simulink model "wireless_dynamic21aMATLAB"  (R2021a)
settings: Solver=FixedStepDiscrete  StartTime=0.0  StopTime=0.1  MaxStep=1e-6  RelTol=1e-3
undefined symbols (not defined in the file): DiscIntNeverNeededParam, Ion, Lithium
libraries: spsSeriesRLCBranchLib x4, spsDiodeLib x4, spsIGBTDiodeLib x4, spsCurrentMeasurementLib x2, spsBatteryLib x1, spsGroundLib x1, spsThreePhaseProgrammableVoltageSourceLib x1, spsUniversalBridgeLib x1, spsVoltageMeasurementLib x1, spspowerguiLib x1, spsMultiWindingTransformerLib x1, spsTriangleGeneratorLib x1
settings Model: Creator=Lenovo  LastModifiedBy=SHREYAS.D
settings SolverCC: AlgebraicLoopSolver=LineSearch
settings DataIOCC: ReturnWorkspaceOutputs=off
settings DebuggingCC: AlgebraicLoopMsg=none  ArithmeticOperatorsInVariantConditions=warning
settings SFSimCC: SimUseLocalCustomCode=off  CustomCodeUndefinedFunction=UseInterfaceOnly
settings RTWCC: RTWUseLocalCustomCode=off  DLArmComputeVersion=20.02.1
settings CodeAppCC: StateflowObjectComments=on
settings SimscapeCC: SimscapeNormalizeSystem=off

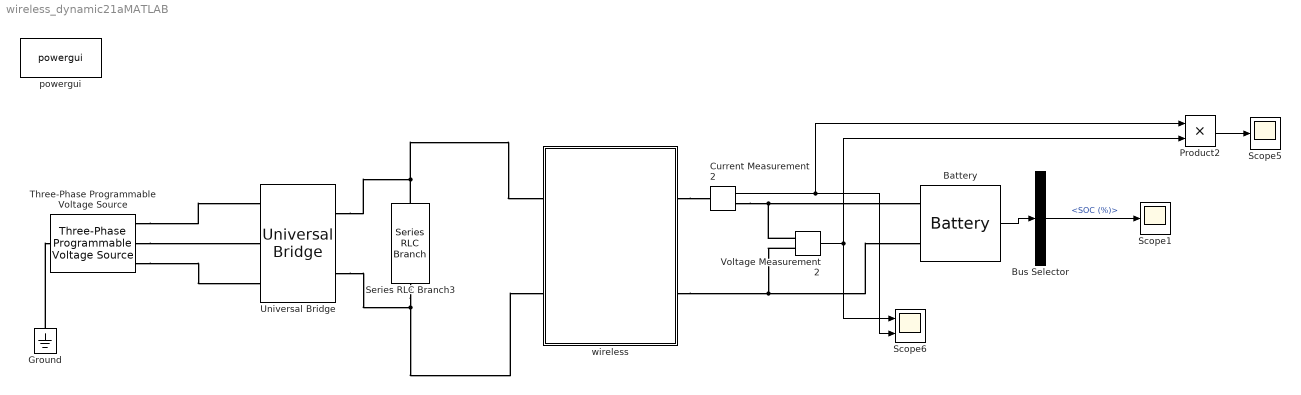
== system wireless_dynamic21aMATLAB ==
  Battery : spsBatteryLib/Battery  BatType=Lithium-Ion  ShowTempParam=off  ThermalPreset=no  ShowAgeParam=off  NomV=60  NomQ=300  SOC=80  Batt_Tr=30  PresetModel=on  MaxQ=300  MinV=45  FullV=69.8392  Dis_rate=130.4348  R=0.002  Normal_OP=271.3043  expZone="[64.8232      14.7391]"  current=[6.5 13 32.5]  Units=Time  Tci=20  NomT=20  T2=-30  MaxQ2=4.8  FullV2=7.1  Normal_OP2=5.655  expZone2="[6.58           1]"  Rca=0.6  ti=2000  Dp=0  Neq0=0  Tsim=1e6  Ta1=25  Qeol=5.4*0.9  Reol=0.013333*1.2  Char_age=[2.3478, 3]  Dis_age=[2.3478, 10]  N1=1500  N2=10500  N3=1000  N4=1400  Ta2=45  N5=950
  Bus Selector : BusSelector  OutputSignals=SOC (%)
  Current Measurement2 : spsCurrentMeasurementLib/Current Measurement  PhasorSimulation=off  OutputType=Complex  PSBequivalent=0
  Ground : spsGroundLib/Ground  LConnTagsString=a
  Product2 : Product
  Scope1 : Scope
  Scope5 : Scope
  Scope6 : Scope  NumInputPorts=2
  Series RLC Branch3 : spsSeriesRLCBranchLib/Series RLC Branch  LConnTagsString=__new0  RConnTagsString=__new0  BranchType=C  Resistance=0.001  Inductance=1e-3  SetiL0=off  InitialCurrent=0  Capacitance=2000e-6  Setx0=off  InitialVoltage=90  Measurements=None
  Three-Phase Programmable Voltage Source : spsThreePhaseProgrammableVoltageSourceLib/Three-Phase Programmable Voltage Source  PositiveSequence="[440  0 50]"  VariationEntity=None  VariationType=Table of time-amplitude pairs  VariationTypeAlt=Step  VariationStep=0.5  VariationRate=10  VariationMagnitude=0.3  VariationFrequency=2  VariationTiming=[1 2]  VariationPhaseA=off  Amplitudes=[1 0.8 1.2 1.0]  TimeValues=[0 0.1 0.15 0.2]  HarmonicGeneration=off  HarmonicA=[3 0.2 -25 0]  HarmonicB=[2 0.15 35 2]  Timing="[0.05  3]"  BusType=swing  Pref=0  Qref=0  Qmin=-inf  Qmax=inf
  Universal Bridge : spsUniversalBridgeLib/Universal Bridge  Arms=3  SnubberResistance=1e5  SnubberCapacitance=inf  Device=Diodes  Ron=1e-3  Lon=0  ForwardVoltages="[  0  0  ]"  ForwardVoltage=0  GTOparameters=[ 10e-6 , 20e-6 ]  IGBTparameters=[ 1e-6 , 2e-6 ]  Measurements=None  Measurements_2=None  converterType=Rectifier
  Voltage Measurement2 : spsVoltageMeasurementLib/Voltage Measurement  PhasorSimulation=off  OutputType=Complex  PSBequivalent=0
  powergui : spspowerguiLib/powergui  Priority=1  SimulationMode=Discrete  SampleTime=1e-6  frequency=60  Iterations=50  frequencyindice=0  Pbase=100e6  ErrMax=1e-4  UnitsV=kV  UnitsW=MW  buscounter=0  FunctionMessages=off  echomessages=off  EnableUseOfTLC=off  CurrentSourceSwitches=off  DisableSnubberDevices=off  DisableRonSwitches=off  DisableVfSwitches=off  DisplayEquations=off  AutomaticDiscreteSolvers=off  SolverType=Tustin/Backward Euler (TBE)  Interpol=off  ExternalGateDelay=off  methode=off  Ts=100  x0status=blocks  SPID=on  SwTol=0  HookPort=off  NonlinearTolerance=1e-4  nMaxIteration=100  ContinueOnMaxIteration=off  RestoreLinks=warning  ResistiveCurrentMeasurement=off  Frange=[0:2:500]  Ylog=off  Xlog=on  ShowGrid=off  save=off  variable=ZData  structure=0  ZoomFFT=off  StartTime=0.0  cycles=1  DisplayStyle=1  fundamental=60  FreqAxis=off  MaxFrequency=1000  frequencyindicesteady=1  RmsSteady=1  display=off
  wireless : Subsystem
  wires:
  Battery/1 -> Bus Selector/1
  Bus Selector/1 -> Scope1/1  "<SOC (%)>"
  Product2/1 -> Scope5/1
  Current Measurement2/1 -> Scope6/2, Product2/1
  Voltage Measurement2/1 -> Scope6/1, Product2/2
  connections:
  wireless/RConn2 -- Voltage Measurement2/LConn2 -- Battery/LConn2
  wireless/RConn1 -- Current Measurement2/LConn1
  Current Measurement2/RConn1 -- Voltage Measurement2/LConn1 -- Battery/LConn1
  Universal Bridge/RConn1 -- wireless/LConn1 -- Series RLC Branch3/LConn1
  Universal Bridge/RConn2 -- wireless/LConn2 -- Series RLC Branch3/RConn1
  Three-Phase Programmable Voltage Source/RConn1 -- Universal Bridge/LConn1
  Three-Phase Programmable Voltage Source/RConn2 -- Universal Bridge/LConn2
  Three-Phase Programmable Voltage Source/RConn3 -- Universal Bridge/LConn3
  Ground/LConn1 -- Three-Phase Programmable Voltage Source/LConn1

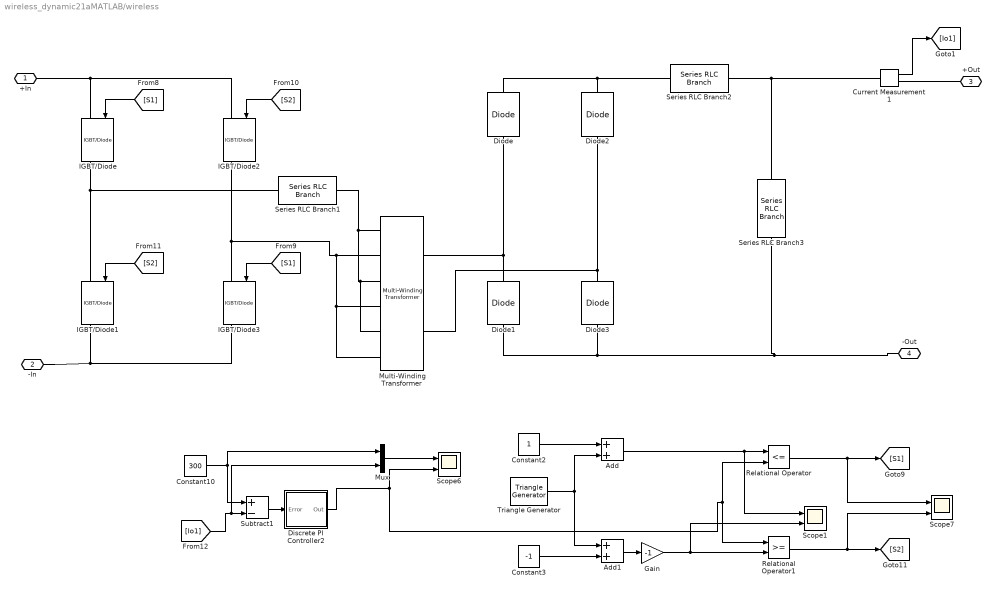
== system wireless_dynamic21aMATLAB/wireless ==
  Add : Sum
  Add1 : Sum
  Constant10 : Constant  Value=300
  Constant2 : Constant
  Constant3 : Constant  Value=-1
  Current Measurement1 : spsCurrentMeasurementLib/Current Measurement  PhasorSimulation=off  OutputType=Complex  PSBequivalent=0
  Diode{,1..3} (4 alike) : spsDiodeLib/Diode  Ron=0.001  Lon=0  Vf=0.8  IC=0  UseSnubber=0  Rs=500  Cs=250e-9  Measurements=off
  Discrete PI Controller2 : Subsystem  AncestorBlock=|  DialogController=POWERSYS.PowerSysDialog  mask(Discrete PI Controller){Kp=0.2, Ki=0.2, Par_Limits=[0.81 0], Init=0, Ts=1e-6}
      | powerlib_extras/Discrete 
      | Control Blocks/Discrete
      | PI Controller
      mask prompts: Kp "Proportional gain (Kp):"; Ki "Integral gain (Ki):"; Par_Limits "Output limits: [ Upper   Lower ]"; Init "Output initial value:"; Ts "Sample time:"
      mask help: This block implements a discrete PI controller.
      mask init:
      | UpperLimit=Par_Limits(1);
      | LowerLimit=Par_Limits(2);
      | power_initmask();
      mask Help: This block is part of a subset of blocks in the Extras library that does not have documentation associated with it, other than the block mask description.
      mask Display: disp('PI');
  Gain : Gain  Gain=-1
  IGBT/Diode{,1..3} (4 alike) : spsIGBTDiodeLib/IGBT//Diode  Ron=1e-3  Rs=1e5  Cs=inf  Measurements=on
  Multi-Winding Transformer : spsMultiWindingTransformerLib/Multi-Winding Transformer  LeftWindings=3  RightWindings=1  TappedWindings=no taps  NumberOfTaps=2  SetSaturation=off  Hysteresis=off  DataFile='hysteresis.mat'  Measurements=None  UNITS=SI  NominalPower=[20e3 20000]  NominalVoltages="[ 600  100  200 120 ]"  WindingResistances=[0.18 0.005 0.005 0.0072]  WindingInductances=[6.1879e-07 1.5915e-07 1.5915e-07 2.2918e-07]  Rm=1800  Lm=0.014324  Saturation=[0 0;0.056566 0.0081028;23.57 0.010264]  BreakLoop=off  DiscreteSolver=Trapezoidal iterative  DataType=on  InitialFlux=0  TransfoNumber=1
      settings: SourceProductBaseCode=PS
  Mux : Mux  Inputs=2
  Relational Operator : RelationalOperator  Operator=<=  OutDataTypeStr=boolean  RndMeth=Simplest
  Relational Operator1 : RelationalOperator  OutDataTypeStr=boolean  RndMeth=Simplest
  Scope1 : Scope  NumInputPorts=2
  Scope6 : Scope  NumInputPorts=2
  Scope7 : Scope  NumInputPorts=2
  Series RLC Branch1 : spsSeriesRLCBranchLib/Series RLC Branch  LConnTagsString=__new0  RConnTagsString=__new0  BranchType=L  Resistance=1  Inductance=0.31e-6  SetiL0=off  InitialCurrent=0  Capacitance=2000000e-6  Setx0=on  InitialVoltage=90  Measurements=None
  Series RLC Branch2 : spsSeriesRLCBranchLib/Series RLC Branch  LConnTagsString=__new0  RConnTagsString=__new0  BranchType=L  Resistance=1  Inductance=6.87e-6  SetiL0=off  InitialCurrent=0  Capacitance=2000000e-6  Setx0=on  InitialVoltage=90  Measurements=None
  Series RLC Branch3 : spsSeriesRLCBranchLib/Series RLC Branch  LConnTagsString=__new0  RConnTagsString=__new0  BranchType=C  Resistance=0.001  Inductance=1e-3  SetiL0=off  InitialCurrent=0  Capacitance=2000e-6  Setx0=off  InitialVoltage=90  Measurements=None
  Subtract1 : Sum  Inputs=+-
  Triangle Generator : spsTriangleGeneratorLib/Triangle Generator  Freq=20e3  Phase=0  Ts=0
  +In : PMIOPort  Side=Left
  -In : PMIOPort  Port=2  Side=Left
  +Out : PMIOPort  Port=3  Side=Right
  -Out : PMIOPort  Port=4  Side=Right
  wires:
  [S1] -> IGBT/Diode3/1
  [S1] -> IGBT/Diode/1
  [S2] -> IGBT/Diode2/1
  [S2] -> IGBT/Diode1/1
  Constant10/1 -> Mux/1, Subtract1/1
  [Io1] -> Subtract1/2, Mux/2
  Subtract1/1 -> Discrete PI Controller2/1(Error)
  Add1/1 -> Gain/1
  Mux/1 -> Scope6/1
  Relational Operator1/1 -> Scope7/2, [S2]
  Relational Operator/1 -> Scope7/1, [S1]
  Discrete PI Controller2/1(Out) -> Relational Operator1/1, Relational Operator/2, Scope6/2
  Add/1 -> Scope1/1, Relational Operator/1
  Triangle Generator/1 -> Add1/1, Add/2
  Constant2/1 -> Add/1
  Constant3/1 -> Add1/2
  Gain/1 -> Scope1/2, Relational Operator1/2
  Current Measurement1/1 -> [Io1]
  connections:
  IGBT/Diode/RConn1 -- IGBT/Diode1/LConn1 -- Series RLC Branch1/LConn1
  IGBT/Diode2/RConn1 -- Multi-Winding Transformer/LConn6 -- Multi-Winding Transformer/LConn4 -- Multi-Winding Transformer/LConn2 -- IGBT/Diode3/LConn1
  IGBT/Diode3/RConn1 -- IGBT/Diode1/RConn1 -- -In/RConn1
  IGBT/Diode2/LConn1 -- +In/RConn1 -- IGBT/Diode/LConn1
  Series RLC Branch1/RConn1 -- Multi-Winding Transformer/LConn5 -- Multi-Winding Transformer/LConn3 -- Multi-Winding Transformer/LConn1
  -Out/RConn1 -- Series RLC Branch3/RConn1 -- Diode3/LConn1 -- Diode1/LConn1
  Diode1/RConn1 -- Diode/LConn1 -- Multi-Winding Transformer/RConn1
  Diode3/RConn1 -- Diode2/LConn1 -- Multi-Winding Transformer/RConn2
  Diode2/RConn1 -- Diode/RConn1 -- Series RLC Branch2/LConn1
  Series RLC Branch2/RConn1 -- Current Measurement1/LConn1 -- Series RLC Branch3/LConn1
  Current Measurement1/RConn1 -- +Out/RConn1

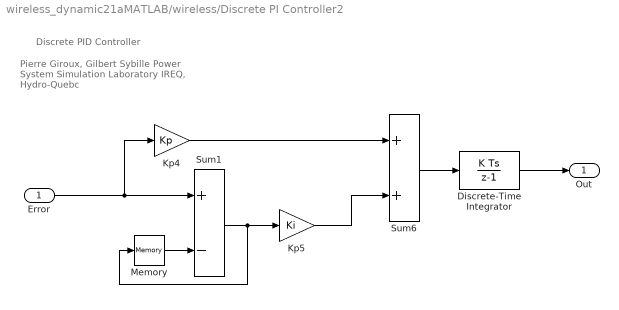
== system wireless_dynamic21aMATLAB/wireless/Discrete PI Controller2 ==
  note: Discrete PID Controller
  note: Pierre Giroux, Gilbert Sybille
      | Power System Simulation Laboratory
      | IREQ, Hydro-Quebc
  Error : Inport  SampleTime=Ts
  Discrete-Time Integrator : DiscreteIntegrator  InitialCondition=Init  SampleTime=Ts  LimitOutput=on  UpperSaturationLimit=UpperLimit  LowerSaturationLimit=LowerLimit  ICPrevOutput=DiscIntNeverNeededParam  ICPrevScaledInput=DiscIntNeverNeededParam
  Kp4 : Gain  Gain=Kp  SaturateOnIntegerOverflow=on  SampleTime=Ts  OutDataTypeStr=Inherit: Same as input  ParamDataTypeStr=Inherit: Same as input
  Kp5 : Gain  Gain=Ki  SaturateOnIntegerOverflow=on  SampleTime=Ts  OutDataTypeStr=Inherit: Same as input  ParamDataTypeStr=Inherit: Same as input
  Memory : Memory
  Sum1 : Sum  Inputs=+-  InputSameDT=on  SaturateOnIntegerOverflow=on  SampleTime=Ts  OutDataTypeStr=Inherit: Same as first input
  Sum6 : Sum  InputSameDT=on  SaturateOnIntegerOverflow=on  SampleTime=Ts  OutDataTypeStr=Inherit: Same as first input
  Out : Outport  SampleTime=Ts  InitialOutput=0
  wires:
  Sum6/1 -> Discrete-Time Integrator/1
  Memory/1 -> Sum1/2
  Sum1/1 -> Kp5/1, Memory/1
  Kp5/1 -> Sum6/2
  Kp4/1 -> Sum6/1
  Discrete-Time Integrator/1 -> Out/1
  Error/1 -> Sum1/1, Kp4/1
